simulink model "UserVehicle_RTW"  (Simulink 10.3)
settings: Solver=ode1  StartTime=0.0  StopTime=inf  FixedStep=0.001  RelTol=1e-3
PreLoadFcn:
  | vehicle = 'Car'; if ~length(which('cmcmd')), cmenv; end
  | UserVehicle_RTW_bus
  | UserVehicle_RTW_params
InitFcn:
  | vehicle = 'Car'; if ~length(which('cmcmd')), cmenv; end
  | UserVehicle_RTW_bus
undefined symbols (not defined in the file or in its folder): Car_Bdy1_mass, Car_Steering_i, Car_WhlBaseF, Car_WhlBaseR
libraries: CarMaker4SL x77
(part 3 of 3)

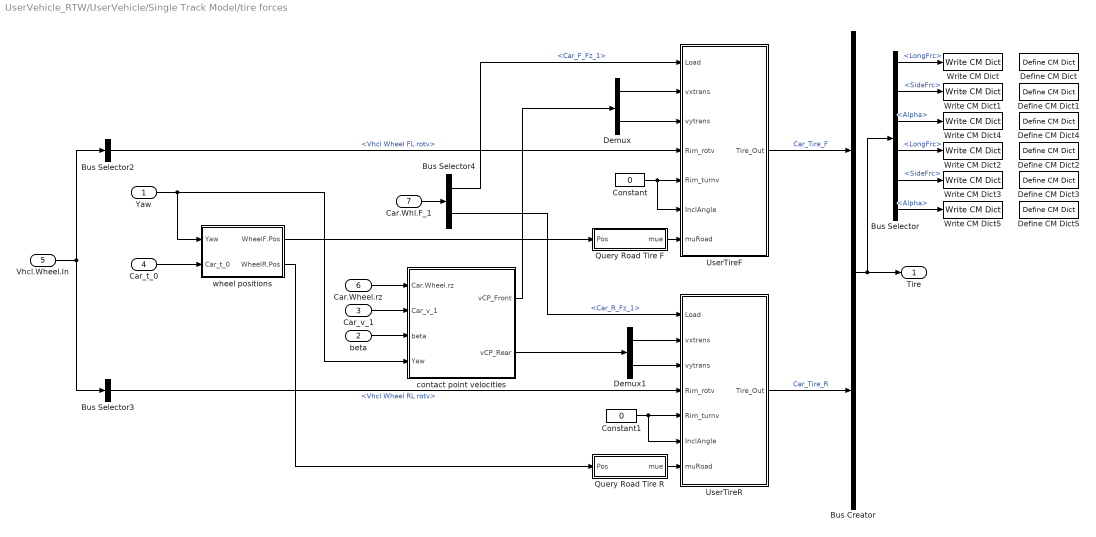
== system UserVehicle_RTW/UserVehicle/Single Track Model/tire forces ==
  Yaw : Inport
  beta : Inport  Port=2
  Car_v_1 : Inport  Port=3
  Car_t_0 : Inport  Port=4
  Vhcl.Wheel.In : Inport  Port=5
  Car.Wheel.rz : Inport  Port=6
  Car.Whl.F_1 : Inport  Port=7
  Bus Creator : BusCreator  Inputs=2
  Bus Selector : BusSelector  OutputSignals=Car_Tire_F.LongFrc,Car_Tire_F.SideFrc,Car_Tire_F.Alpha,Car_Tire_R.LongFrc,Car_Tire_R.SideFrc,Car_Tire_R.Alpha
  Bus Selector2 : BusSelector  OutputSignals=Vhcl Wheel FL rotv
  Bus Selector3 : BusSelector  OutputSignals=Vhcl Wheel RL rotv
  Bus Selector4 : BusSelector  OutputSignals=Car_F_Fz_1,Car_R_Fz_1
  Constant : Constant  Value=0
  Constant1 : Constant  Value=0
  Define CM Dict : CarMaker4SL/Define CM Dict  xname=Tire.F.LongFrc  xunit=N  xmono=off  xtype=Double4  xdvaplace=None  xnstates=0  xfirststate=0  xinitial=0
  Define CM Dict1 : CarMaker4SL/Define CM Dict  xname=Tire.F.SideFrc  xunit=N  xmono=off  xtype=Double4  xdvaplace=None  xnstates=0  xfirststate=0  xinitial=0
  Define CM Dict2 : CarMaker4SL/Define CM Dict  xname=Tire.R.LongFrc  xunit=N  xmono=off  xtype=Double4  xdvaplace=None  xnstates=0  xfirststate=0  xinitial=0
  Define CM Dict3 : CarMaker4SL/Define CM Dict  xname=Tire.R.SideFrc  xunit=N  xmono=off  xtype=Double4  xdvaplace=None  xnstates=0  xfirststate=0  xinitial=0
  Define CM Dict4 : CarMaker4SL/Define CM Dict  xname=Tire.F.Alpha  xunit=rad  xmono=off  xtype=Double4  xdvaplace=None  xnstates=0  xfirststate=0  xinitial=0
  Define CM Dict5 : CarMaker4SL/Define CM Dict  xname=Tire.R.Alpha  xunit=rad  xmono=off  xtype=Double4  xdvaplace=None  xnstates=0  xfirststate=0  xinitial=0
  Demux : Demux  Outputs=2
  Demux1 : Demux  Outputs=2
  Query Road Tire F : Subsystem
  Query Road Tire R : Subsystem
  UserTireF : Subsystem
  UserTireR : Subsystem
  Write CM Dict : CarMaker4SL/Write CM Dict  xname=Tire.F.LongFrc  xsync=off
  Write CM Dict1 : CarMaker4SL/Write CM Dict  xname=Tire.F.SideFrc  xsync=off
  Write CM Dict2 : CarMaker4SL/Write CM Dict  xname=Tire.R.LongFrc  xsync=off
  Write CM Dict3 : CarMaker4SL/Write CM Dict  xname=Tire.R.SideFrc  xsync=off
  Write CM Dict4 : CarMaker4SL/Write CM Dict  xname=Tire.F.Alpha  xsync=off
  Write CM Dict5 : CarMaker4SL/Write CM Dict  xname=Tire.R.Alpha  xsync=off
  contact point velocities : Subsystem
  wheel positions : Subsystem
  Tire : Outport  VectorParamsAs1DForOutWhenUnconnected=off
  wires:
  Bus Selector/6 -> Write CM Dict5/1  "<Alpha>"
  Bus Selector/3 -> Write CM Dict4/1  "<Alpha>"
  Bus Selector/5 -> Write CM Dict3/1  "<SideFrc>"
  Bus Selector/4 -> Write CM Dict2/1  "<LongFrc>"
  Bus Selector/2 -> Write CM Dict1/1  "<SideFrc>"
  Bus Selector/1 -> Write CM Dict/1  "<LongFrc>"
  Demux1/2 -> UserTireR/3(vytrans)
  Demux/2 -> UserTireF/3(vytrans)
  Bus Creator/1 -> Bus Selector/1, Tire/1
  Bus Selector4/1 -> UserTireF/1(Load)  "<Car_F_Fz_1>"
  Car.Whl.F_1/1 -> Bus Selector4/1
  Bus Selector4/2 -> UserTireR/1(Load)  "<Car_R_Fz_1>"
  contact point velocities/2(vCP_Rear) -> Demux1/1
  Demux1/1 -> UserTireR/2(vxtrans)
  Demux/1 -> UserTireF/2(vxtrans)
  contact point velocities/1(vCP_Front) -> Demux/1
  Car.Wheel.rz/1 -> contact point velocities/1(Car.Wheel.rz)
  beta/1 -> contact point velocities/3(beta)
  Car_v_1/1 -> contact point velocities/2(Car_v_1)
  Constant/1 -> UserTireF/5(Rim_turnv), UserTireF/6(InclAngle)
  Bus Selector3/1 -> UserTireR/4(Rim_rotv)  "<Vhcl Wheel RL rotv>"
  wheel positions/2(WheelR.Pos) -> Query Road Tire R/1(Pos)
  wheel positions/1(WheelF.Pos) -> Query Road Tire F/1(Pos)
  Car_t_0/1 -> wheel positions/2(Car_t_0)
  Yaw/1 -> contact point velocities/4(Yaw), wheel positions/1(Yaw)
  Query Road Tire R/1(mue) -> UserTireR/7(muRoad)
  Query Road Tire F/1(mue) -> UserTireF/7(muRoad)
  Bus Selector2/1 -> UserTireF/4(Rim_rotv)  "<Vhcl Wheel FL rotv>"
  Vhcl.Wheel.In/1 -> Bus Selector3/1, Bus Selector2/1
  Constant1/1 -> UserTireR/6(InclAngle), UserTireR/5(Rim_turnv)
  UserTireR/1(Tire_Out) -> Bus Creator/2  "Car_Tire_R"
  UserTireF/1(Tire_Out) -> Bus Creator/1  "Car_Tire_F"

== system UserVehicle_RTW/UserVehicle/Single Track Model/vehicle motion ==
  Car.Whl.F_1 : Inport
  Car.Beta : Inport  Port=2
  Car_Yaw : Inport  Port=3
  global frame : Subsystem
  vehicle frame : Subsystem
  Car.a_1 : Outport  VectorParamsAs1DForOutWhenUnconnected=off
  Car.v_1 : Outport  Port=2  VectorParamsAs1DForOutWhenUnconnected=off
  Car.a_0 : Outport  Port=3  VectorParamsAs1DForOutWhenUnconnected=off
  Car.v_0 : Outport  Port=4  VectorParamsAs1DForOutWhenUnconnected=off
  Car_t_0 : Outport  Port=5  VectorParamsAs1DForOutWhenUnconnected=off
  Car.Dist : Outport  Port=6  VectorParamsAs1DForOutWhenUnconnected=off
  wires:
  global frame/3(Car.t_0) -> Car_t_0/1
  global frame/2(Car_v_0) -> Car.v_0/1
  global frame/1(Car.a_0) -> Car.a_0/1
  Car.Beta/1 -> vehicle frame/2(Car.Beta)
  Car.Whl.F_1/1 -> vehicle frame/1(Car.Whl.F_1)
  vehicle frame/2(Car.v_1) -> global frame/2(Car.v_1), Car.v_1/1
  vehicle frame/1(Car.a_1) -> global frame/1(Car.a_1), Car.a_1/1
  Car_Yaw/1 -> global frame/3(Car.Yaw)
  vehicle frame/3(Car.Dist) -> Car.Dist/1

== system UserVehicle_RTW/UserVehicle/Single Track Model/wheel torques ==
  WheelTrq_1 : Inport
  Add : Sum  Inputs=+-
  Add1 : Sum  Inputs=+-
  Bus Creator : BusCreator  Inputs=2
  Bus Selector1 : BusSelector  OutputSignals=Car_Tire_F.RollResist,Car_Tire_F.LongFrc,Car_Tire_F.rBelt_eff
  Bus Selector2 : BusSelector  OutputSignals=Car_Tire_R.RollResist,Car_Tire_R.LongFrc,Car_Tire_R.rBelt_eff
  Product : Product  RndMeth=Zero
  Product1 : Product  RndMeth=Zero
  Car.Trq2W : Outport  VectorParamsAs1DForOutWhenUnconnected=off
  wires:
  Add1/1 -> Bus Creator/2  "Trq_R"
  Product1/1 -> Add1/2
  Bus Selector2/3 -> Product1/2  "<rBelt_eff>"
  Bus Selector2/2 -> Product1/1  "<LongFrc>"
  Bus Selector2/1 -> Add1/1  "<RollResist>"
  Add/1 -> Bus Creator/1  "Trq_F"
  Product/1 -> Add/2
  Bus Selector1/3 -> Product/2  "<rBelt_eff>"
  Bus Selector1/2 -> Product/1  "<LongFrc>"
  Bus Selector1/1 -> Add/1  "<RollResist>"
  WheelTrq_1/1 -> Bus Selector2/1, Bus Selector1/1
  Bus Creator/1 -> Car.Trq2W/1

== system UserVehicle_RTW/UserVehicle/Single Track Model/yaw ==
  WheelFrc_1 : Inport
  1/ J : Gain  Gain=1/1322.5  SaturateOnIntegerOverflow=on  OutDataTypeStr=Inherit: Same as input  ParamDataTypeStr=Inherit: Same as input
  Bus Creator : BusCreator  Inputs=3
  Bus Selector : BusSelector  OutputSignals=Vhcl Cfg Yaw
  Bus Selector1 : BusSelector  OutputSignals=Car_F_Fy_1,Car_R_Fy_1
  Multiply : Product  Inputs=**  OutDataTypeStr=double
  "S_F * l_F " : Product  InputSameDT=on  SaturateOnIntegerOverflow=on  OutDataTypeStr=Inherit: Same as first input
  "S_R * l_R " : Product  InputSameDT=on  SaturateOnIntegerOverflow=on  OutDataTypeStr=Inherit: Same as first input
  Sum : Sum  Inputs=+-  InputSameDT=on  SaturateOnIntegerOverflow=on  OutDataTypeStr=Inherit: Same as first input
  Vehicle Initial Cfg : CarMaker4SL/Vehicle Initial Cfg
      settings: SourceProductName=CarMaker4SL
  aYaw * dt : Integrator  ExternalReset=level
  l__F : Constant  Value=Car_WhlBaseF
  l__R : Constant  Value=-Car_WhlBaseR
  vYaw * dt : Integrator  ExternalReset=level  InitialConditionSource=external
  Car.Yaw : Outport  VectorParamsAs1DForOutWhenUnconnected=off
  wires:
  Bus Selector1/2 -> "S_R * l_R "/1  "<Car_R_Fy_1>"
  Bus Selector1/1 -> "S_F * l_F "/1  "<Car_F_Fy_1>"
  WheelFrc_1/1 -> Bus Selector1/1
  Bus Creator/1 -> Car.Yaw/1
  "S_R * l_R "/1 -> Sum/2
  l__R/1 -> "S_R * l_R "/2
  "S_F * l_F "/1 -> Sum/1
  l__F/1 -> "S_F * l_F "/2
  Bus Selector/1 -> vYaw * dt/3  "<Vhcl Cfg Yaw>"
  Sum/1 -> 1/ J/1
  1/ J/1 -> Bus Creator/3, aYaw * dt/1  "Yawpp"
  vYaw * dt/1 -> Bus Creator/1  "Yaw"
  Multiply/1 -> Bus Creator/2, vYaw * dt/1  "Yawp"
  [TRStart] -> aYaw * dt/2, vYaw * dt/2
  aYaw * dt/1 -> Multiply/2
  [TRSim] -> Multiply/1
  Vehicle Initial Cfg/1 -> Bus Selector/1

== system UserVehicle_RTW/UserVehicle/CreateBus Vhcl.Fr1/Tr2Fr0/Subsystem_00 ==
  sincos : Inport
  Bus Selector : BusSelector  OutputSignals=cry,crz
  Product : Product  RndMeth=Zero
  Tr2Fr1_00 : Outport  VectorParamsAs1DForOutWhenUnconnected=off
  wires:
  Bus Selector/2 -> Product/2  "<crz>"
  Bus Selector/1 -> Product/1  "<cry>"
  Product/1 -> Tr2Fr1_00/1
  sincos/1 -> Bus Selector/1

== system UserVehicle_RTW/UserVehicle/CreateBus Vhcl.Fr1/Tr2Fr0/Subsystem_01 ==
  sincos : Inport
  Add : Sum  Inputs=+-
  Bus Selector : BusSelector  OutputSignals=srx,sry,crz,crx,srz
  Product : Product  Inputs=3  RndMeth=Zero
  Product1 : Product  RndMeth=Zero
  Tr2Fr1_01 : Outport  VectorParamsAs1DForOutWhenUnconnected=off
  wires:
  Bus Selector/5 -> Product1/2  "<srz>"
  Bus Selector/4 -> Product1/1  "<crx>"
  Bus Selector/3 -> Product/3  "<crz>"
  Bus Selector/2 -> Product/2  "<sry>"
  Bus Selector/1 -> Product/1  "<srx>"
  Add/1 -> Tr2Fr1_01/1
  Product1/1 -> Add/2
  Product/1 -> Add/1
  sincos/1 -> Bus Selector/1

== system UserVehicle_RTW/UserVehicle/CreateBus Vhcl.Fr1/Tr2Fr0/Subsystem_02 ==
  sincos : Inport
  Add : Sum
  Bus Selector : BusSelector  OutputSignals=crx,sry,crz,srx,srz
  Product : Product  Inputs=3  RndMeth=Zero
  Product1 : Product  RndMeth=Zero
  Tr2Fr1_02 : Outport  VectorParamsAs1DForOutWhenUnconnected=off
  wires:
  Bus Selector/4 -> Product1/1  "<srx>"
  Bus Selector/5 -> Product1/2  "<srz>"
  Bus Selector/3 -> Product/3  "<crz>"
  Bus Selector/2 -> Product/2  "<sry>"
  Bus Selector/1 -> Product/1  "<crx>"
  sincos/1 -> Bus Selector/1
  Product/1 -> Add/1
  Product1/1 -> Add/2
  Add/1 -> Tr2Fr1_02/1

== system UserVehicle_RTW/UserVehicle/CreateBus Vhcl.Fr1/Tr2Fr0/Subsystem_10 ==
  sincos : Inport
  Bus Selector : BusSelector  OutputSignals=cry,srz
  Product : Product  RndMeth=Zero
  Tr2Fr1_10 : Outport  VectorParamsAs1DForOutWhenUnconnected=off
  wires:
  sincos/1 -> Bus Selector/1
  Product/1 -> Tr2Fr1_10/1
  Bus Selector/1 -> Product/1  "<cry>"
  Bus Selector/2 -> Product/2  "<srz>"

== system UserVehicle_RTW/UserVehicle/CreateBus Vhcl.Fr1/Tr2Fr0/Subsystem_11 ==
  sincos : Inport
  Add : Sum
  Bus Selector : BusSelector  OutputSignals=srx,sry,srz,crx,crz
  Product : Product  Inputs=3  RndMeth=Zero
  Product1 : Product  RndMeth=Zero
  Tr2Fr1_11 : Outport  VectorParamsAs1DForOutWhenUnconnected=off
  wires:
  Bus Selector/4 -> Product1/1  "<crx>"
  Bus Selector/5 -> Product1/2  "<crz>"
  Bus Selector/3 -> Product/3  "<srz>"
  Bus Selector/2 -> Product/2  "<sry>"
  Bus Selector/1 -> Product/1  "<srx>"
  Add/1 -> Tr2Fr1_11/1
  Product1/1 -> Add/2
  Product/1 -> Add/1
  sincos/1 -> Bus Selector/1

== system UserVehicle_RTW/UserVehicle/CreateBus Vhcl.Fr1/Tr2Fr0/Subsystem_12 ==
  sincos : Inport
  Add : Sum  Inputs=+-
  Bus Selector : BusSelector  OutputSignals=crx,sry,srz,srx,crz
  Product : Product  Inputs=3  RndMeth=Zero
  Product1 : Product  RndMeth=Zero
  Tr2Fr1_12 : Outport  VectorParamsAs1DForOutWhenUnconnected=off
  wires:
  Bus Selector/4 -> Product1/1  "<srx>"
  Bus Selector/5 -> Product1/2  "<crz>"
  Bus Selector/3 -> Product/3  "<srz>"
  Bus Selector/2 -> Product/2  "<sry>"
  Bus Selector/1 -> Product/1  "<crx>"
  sincos/1 -> Bus Selector/1
  Product/1 -> Add/1
  Product1/1 -> Add/2
  Add/1 -> Tr2Fr1_12/1

== system UserVehicle_RTW/UserVehicle/CreateBus Vhcl.Fr1/Tr2Fr0/Subsystem_20 ==
  sincos : Inport
  Bus Selector : BusSelector  OutputSignals=sry
  Gain : Gain  Gain=-1
  Tr2Fr1_20 : Outport  VectorParamsAs1DForOutWhenUnconnected=off
  wires:
  Bus Selector/1 -> Gain/1  "<sry>"
  Gain/1 -> Tr2Fr1_20/1
  sincos/1 -> Bus Selector/1

== system UserVehicle_RTW/UserVehicle/CreateBus Vhcl.Fr1/Tr2Fr0/Subsystem_21 ==
  sincos : Inport
  Bus Selector : BusSelector  OutputSignals=srx,cry
  Product : Product  RndMeth=Zero
  Tr2Fr1_21 : Outport  VectorParamsAs1DForOutWhenUnconnected=off
  wires:
  Bus Selector/2 -> Product/2  "<cry>"
  Bus Selector/1 -> Product/1  "<srx>"
  Product/1 -> Tr2Fr1_21/1
  sincos/1 -> Bus Selector/1

== system UserVehicle_RTW/UserVehicle/CreateBus Vhcl.Fr1/Tr2Fr0/Subsystem_22 ==
  sincos : Inport
  Bus Selector : BusSelector  OutputSignals=crx,cry
  Product : Product  RndMeth=Zero
  Tr2Fr1_22 : Outport  VectorParamsAs1DForOutWhenUnconnected=off
  wires:
  Bus Selector/2 -> Product/2  "<cry>"
  Bus Selector/1 -> Product/1  "<crx>"
  sincos/1 -> Bus Selector/1
  Product/1 -> Tr2Fr1_22/1

== system UserVehicle_RTW/UserVehicle/CreateBus Vhcl.Fr1/Tr2Fr0/sincos ==
  Car : Inport
  Bus Creator : BusCreator  Inputs=6
  Bus Selector : BusSelector  OutputSignals=Road_Fr1_rx,Road_Fr1_ry,Car_Yaw.Yaw
  Trigonometric Function : Trigonometry
  Trigonometric Function1 : Trigonometry  Operator=cos
  Trigonometric Function2 : Trigonometry
  Trigonometric Function3 : Trigonometry
  Trigonometric Function4 : Trigonometry  Operator=cos
  Trigonometric Function5 : Trigonometry  Operator=cos
  sincos : Outport  VectorParamsAs1DForOutWhenUnconnected=off
  wires:
  Bus Creator/1 -> sincos/1
  Trigonometric Function/1 -> Bus Creator/1  "srx"
  Trigonometric Function3/1 -> Bus Creator/2  "sry"
  Trigonometric Function2/1 -> Bus Creator/3  "srz"
  Trigonometric Function1/1 -> Bus Creator/4  "crx"
  Trigonometric Function4/1 -> Bus Creator/5  "cry"
  Trigonometric Function5/1 -> Bus Creator/6  "crz"
  Car/1 -> Bus Selector/1
  Bus Selector/3 -> Trigonometric Function5/1, Trigonometric Function2/1  "<Yaw>"
  Bus Selector/2 -> Trigonometric Function4/1, Trigonometric Function3/1  "<Road_Fr1_ry>"
  Bus Selector/1 -> Trigonometric Function1/1, Trigonometric Function/1  "<Road_Fr1_rx>"

== system UserVehicle_RTW/UserVehicle/Single Track Model/Tire2Wheel/Fr12Fr0_2D ==
  rz : Inport
  x_1 : Inport  Port=2
  y_1 : Inport  Port=3
  Add : Sum  Inputs=+-
  Add1 : Sum
  Demux : Demux  Outputs=2
  Demux1 : Demux  Outputs=2
  Mux : Mux  Inputs=2
  Product : Product  RndMeth=Zero
  Product1 : Product  RndMeth=Zero
  Trigonometric Function : Trigonometry  Operator=cos
  Trigonometric Function1 : Trigonometry
  x_0 : Outport  VectorParamsAs1DForOutWhenUnconnected=off
  y_0 : Outport  Port=2  VectorParamsAs1DForOutWhenUnconnected=off
  wires:
  Trigonometric Function/1 -> Product/1
  Trigonometric Function1/1 -> Product1/1
  Add/1 -> x_0/1
  Add1/1 -> y_0/1
  rz/1 -> Trigonometric Function1/1, Trigonometric Function/1
  x_1/1 -> Mux/1
  y_1/1 -> Mux/2
  Mux/1 -> Product1/2, Product/2
  Product/1 -> Demux/1
  Demux/1 -> Add/1  "x*cos(rz)"
  Product1/1 -> Demux1/1
  Demux1/2 -> Add/2  "y*sin(rz)"
  Demux/2 -> Add1/1  "y*cos(rz)"
  Demux1/1 -> Add1/2  "x*sin(rz)"

== system UserVehicle_RTW/UserVehicle/Single Track Model/sideslip angle/Subsystem ==
  vYaw : Inport
  v : Inport  Port=2
  In3 : Inport  Port=3
  If : If  IfExpression=u1 ~= 0
  If Action Subsystem : Subsystem  TreatAsAtomicUnit=on
  If Action Subsystem1 : Subsystem  TreatAsAtomicUnit=on
  Merge : Merge
  Sum1 : Sum  Inputs=-+  InputSameDT=on  SaturateOnIntegerOverflow=on  OutDataTypeStr=Inherit: Same as first input
  Out1 : Outport  VectorParamsAs1DForOutWhenUnconnected=off
  wires:
  vYaw/1 -> Sum1/1
  v/1 -> If Action Subsystem/1(v), If/1
  Sum1/1 -> Out1/1
  If Action Subsystem/1(Out1) -> Merge/1
  If Action Subsystem1/1(Out1) -> Merge/2
  Merge/1 -> Sum1/2
  If/2 -> If Action Subsystem1/Action
  In3/1 -> If Action Subsystem/2(In3)
  If/1 -> If Action Subsystem/Action

== system UserVehicle_RTW/UserVehicle/Single Track Model/tire forces/Query Road Tire F ==
  Pos : Inport
  Constant1 : Constant  Value=0
  Constant2 : Constant  Value=0
  Define CM Dict1 : CarMaker4SL/Define CM Dict  xname=Tire.F.mue  xmono=off  xtype=Double4  xdvaplace=None  xnstates=0  xfirststate=0  xinitial=0
  Demux : Demux  Outputs=2
  Memory : Memory
  Mux : Mux  Inputs=3
  Subsystem : Subsystem
  Write CM Dict1 : CarMaker4SL/Write CM Dict  xname=Tire.F.mue  xsync=off
  mue : Outport  VectorParamsAs1DForOutWhenUnconnected=off
  wires:
  Constant1/1 -> Subsystem/3(Side)
  [TRSim] -> Subsystem/Enable
  Pos/1 -> Demux/1
  Memory/1 -> Subsystem/2(Dist)
  Demux/1 -> Mux/1
  Demux/2 -> Mux/2
  Mux/1 -> Subsystem/1(xyz)
  Subsystem/2(Dist Out) -> Memory/1
  Subsystem/1(Fric) -> Write CM Dict1/1, mue/1
  Constant2/1 -> Mux/3

== system UserVehicle_RTW/UserVehicle/Single Track Model/tire forces/Query Road Tire R ==
  Pos : Inport
  Constant1 : Constant  Value=0
  Constant2 : Constant  Value=0
  Define CM Dict1 : CarMaker4SL/Define CM Dict  xname=Tire.R.mue  xmono=off  xtype=Double4  xdvaplace=None  xnstates=0  xfirststate=0  xinitial=0
  Demux : Demux  Outputs=2
  Memory : Memory
  Mux : Mux  Inputs=3
  Subsystem : Subsystem
  Write CM Dict1 : CarMaker4SL/Write CM Dict  xname=Tire.R.mue  xsync=off
  mue : Outport  VectorParamsAs1DForOutWhenUnconnected=off
  wires:
  [TRSim] -> Subsystem/Enable
  Constant2/1 -> Mux/3
  Subsystem/1(Fric) -> Write CM Dict1/1, mue/1
  Subsystem/2(Dist Out) -> Memory/1
  Mux/1 -> Subsystem/1(xyz)
  Demux/2 -> Mux/2
  Demux/1 -> Mux/1
  Constant1/1 -> Subsystem/3(Side)
  Memory/1 -> Subsystem/2(Dist)
  Pos/1 -> Demux/1

== system UserVehicle_RTW/UserVehicle/Single Track Model/tire forces/UserTireF ==
  Load : Inport
  vxtrans : Inport  Port=2
  vytrans : Inport  Port=3
  Rim_rotv : Inport  Port=4
  Rim_turnv : Inport  Port=5
  InclAngle : Inport  Port=6
  muRoad : Inport  Port=7
  Bus Creator3 : BusCreator  Inputs=11
  UserTire : S-Function  FunctionName=tire_lin  SFunctionDeploymentMode=off  EnableBusSupport=off
  Tire_Out : Outport  VectorParamsAs1DForOutWhenUnconnected=off
  wires:
  UserTire/8 -> Bus Creator3/8  "LoadFrc"
  UserTire/7 -> Bus Creator3/7  "SideFrc"
  UserTire/6 -> Bus Creator3/6  "LongFrc"
  UserTire/5 -> Bus Creator3/5  "vBelt"
  UserTire/4 -> Bus Creator3/4  "rBelt_eff"
  UserTire/3 -> Bus Creator3/3  "TurnSlp"
  UserTire/2 -> Bus Creator3/2  "Alpha"
  UserTire/1 -> Bus Creator3/1  "Slp"
  Bus Creator3/1 -> Tire_Out/1
  Load/1 -> UserTire/1
  vxtrans/1 -> UserTire/2
  vytrans/1 -> UserTire/3
  Rim_rotv/1 -> UserTire/4
  InclAngle/1 -> UserTire/6
  muRoad/1 -> UserTire/7
  Rim_turnv/1 -> UserTire/5
  UserTire/9 -> Bus Creator3/9  "OverturnTrq"
  UserTire/10 -> Bus Creator3/10  "RollResist"
  UserTire/11 -> Bus Creator3/11  "AlignTrq"

== system UserVehicle_RTW/UserVehicle/Single Track Model/tire forces/UserTireR ==
  Load : Inport
  vxtrans : Inport  Port=2
  vytrans : Inport  Port=3
  Rim_rotv : Inport  Port=4
  Rim_turnv : Inport  Port=5
  InclAngle : Inport  Port=6
  muRoad : Inport  Port=7
  Bus Creator3 : BusCreator  Inputs=11
  UserTire : S-Function  FunctionName=tire_lin  SFunctionDeploymentMode=off  EnableBusSupport=off
  Tire_Out : Outport  VectorParamsAs1DForOutWhenUnconnected=off
  wires:
  UserTire/11 -> Bus Creator3/11  "AlignTrq"
  UserTire/10 -> Bus Creator3/10  "RollResist"
  UserTire/9 -> Bus Creator3/9  "OverturnTrq"
  Rim_turnv/1 -> UserTire/5
  muRoad/1 -> UserTire/7
  InclAngle/1 -> UserTire/6
  Rim_rotv/1 -> UserTire/4
  vytrans/1 -> UserTire/3
  vxtrans/1 -> UserTire/2
  Load/1 -> UserTire/1
  Bus Creator3/1 -> Tire_Out/1
  UserTire/1 -> Bus Creator3/1  "Slp"
  UserTire/2 -> Bus Creator3/2  "Alpha"
  UserTire/3 -> Bus Creator3/3  "TurnSlp"
  UserTire/4 -> Bus Creator3/4  "rBelt_eff"
  UserTire/5 -> Bus Creator3/5  "vBelt"
  UserTire/6 -> Bus Creator3/6  "LongFrc"
  UserTire/7 -> Bus Creator3/7  "SideFrc"
  UserTire/8 -> Bus Creator3/8  "LoadFrc"

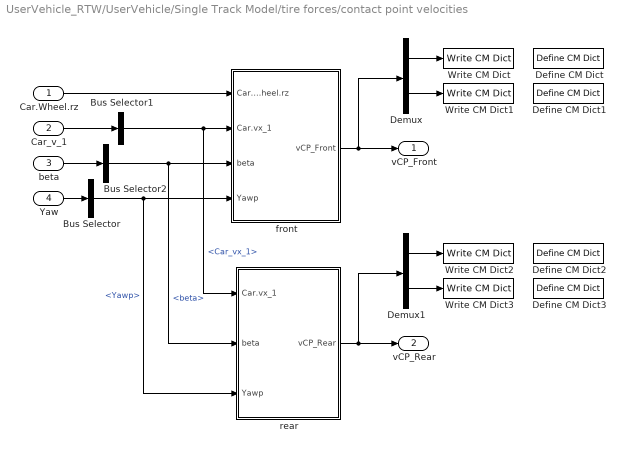
== system UserVehicle_RTW/UserVehicle/Single Track Model/tire forces/contact point velocities ==
  Car.Wheel.rz : Inport
  Car_v_1 : Inport  Port=2
  beta : Inport  Port=3
  Yaw : Inport  Port=4
  Bus Selector : BusSelector  OutputSignals=Yawp
  Bus Selector1 : BusSelector  OutputSignals=Car_vx_1
  Bus Selector2 : BusSelector  OutputSignals=beta
  Define CM Dict : CarMaker4SL/Define CM Dict  xname=Tire.F.vx  xunit=m/s  xmono=off  xtype=Double4  xdvaplace=None  xnstates=0  xfirststate=0  xinitial=0
  Define CM Dict1 : CarMaker4SL/Define CM Dict  xname=Tire.F.vy  xunit=m/s  xmono=off  xtype=Double4  xdvaplace=None  xnstates=0  xfirststate=0  xinitial=0
  Define CM Dict2 : CarMaker4SL/Define CM Dict  xname=Tire.R.vx  xunit=m/s  xmono=off  xtype=Double4  xdvaplace=None  xnstates=0  xfirststate=0  xinitial=0
  Define CM Dict3 : CarMaker4SL/Define CM Dict  xname=Tire.R.vy  xunit=m/s  xmono=off  xtype=Double4  xdvaplace=None  xnstates=0  xfirststate=0  xinitial=0
  Demux : Demux  Outputs=2
  Demux1 : Demux  Outputs=2
  Write CM Dict : CarMaker4SL/Write CM Dict  xname=Tire.F.vx  xsync=off
  Write CM Dict1 : CarMaker4SL/Write CM Dict  xname=Tire.F.vy  xsync=off
  Write CM Dict2 : CarMaker4SL/Write CM Dict  xname=Tire.R.vx  xsync=off
  Write CM Dict3 : CarMaker4SL/Write CM Dict  xname=Tire.R.vy  xsync=off
  front : Subsystem
  rear : Subsystem
  vCP_Front : Outport  VectorParamsAs1DForOutWhenUnconnected=off
  vCP_Rear : Outport  Port=2  VectorParamsAs1DForOutWhenUnconnected=off
  wires:
  Car_v_1/1 -> Bus Selector1/1
  Bus Selector1/1 -> rear/1(Car.vx_1), front/2(Car.vx_1)  "<Car_vx_1>"
  Demux/2 -> Write CM Dict1/1
  Demux/1 -> Write CM Dict/1
  Demux1/2 -> Write CM Dict3/1
  Demux1/1 -> Write CM Dict2/1
  Bus Selector2/1 -> front/3(beta), rear/2(beta)  "<beta>"
  Bus Selector/1 -> rear/3(Yawp), front/4(Yawp)  "<Yawp>"
  Yaw/1 -> Bus Selector/1
  front/1(vCP_Front) -> Demux/1, vCP_Front/1
  Car.Wheel.rz/1 -> front/1(Car.Wheel.rz)
  beta/1 -> Bus Selector2/1
  rear/1(vCP_Rear) -> vCP_Rear/1, Demux1/1

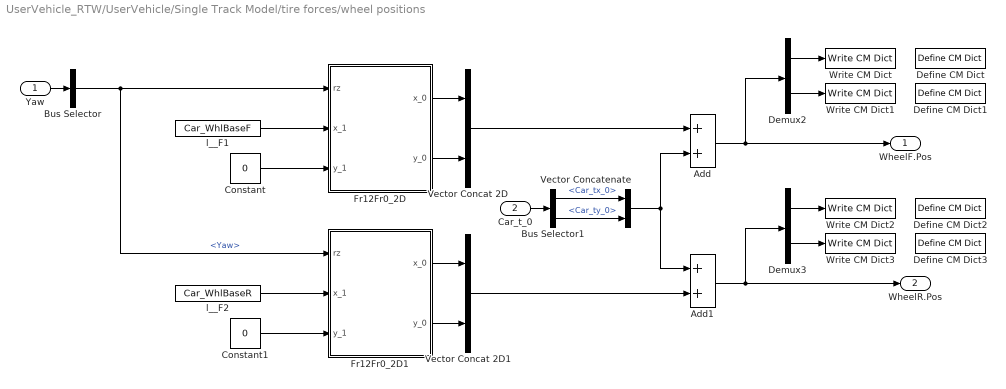
== system UserVehicle_RTW/UserVehicle/Single Track Model/tire forces/wheel positions ==
  Yaw : Inport
  Car_t_0 : Inport  Port=2
  Add : Sum
  Add1 : Sum
  Bus Selector : BusSelector  OutputSignals=Yaw
  Bus Selector1 : BusSelector  OutputSignals=Car_tx_0,Car_ty_0
  Constant : Constant  Value=0
  Constant1 : Constant  Value=0
  Define CM Dict : CarMaker4SL/Define CM Dict  xname=Car.CF.x_0  xunit=m  xmono=off  xtype=Double4  xdvaplace=None  xnstates=0  xfirststate=0  xinitial=0
  Define CM Dict1 : CarMaker4SL/Define CM Dict  xname=Car.CF.y_0  xunit=m  xmono=off  xtype=Double4  xdvaplace=None  xnstates=0  xfirststate=0  xinitial=0
  Define CM Dict2 : CarMaker4SL/Define CM Dict  xname=Car.CR.x_0  xunit=m  xmono=off  xtype=Double4  xdvaplace=None  xnstates=0  xfirststate=0  xinitial=0
  Define CM Dict3 : CarMaker4SL/Define CM Dict  xname=Car.CR.y_0  xunit=m  xmono=off  xtype=Double4  xdvaplace=None  xnstates=0  xfirststate=0  xinitial=0
  Demux2 : Demux  Outputs=2
  Demux3 : Demux  Outputs=2
  Fr12Fr0_2D : Subsystem
  Fr12Fr0_2D1 : Subsystem
  Vector Concat 2D : Concatenate
  Vector Concat 2D1 : Concatenate
  Vector Concatenate : Concatenate
  Write CM Dict : CarMaker4SL/Write CM Dict  xname=Car.CF.x_0  xsync=off
  Write CM Dict1 : CarMaker4SL/Write CM Dict  xname=Car.CF.y_0  xsync=off
  Write CM Dict2 : CarMaker4SL/Write CM Dict  xname=Car.CR.x_0  xsync=off
  Write CM Dict3 : CarMaker4SL/Write CM Dict  xname=Car.CR.y_0  xsync=off
  l__F1 : Constant  Value=Car_WhlBaseF
  l__F2 : Constant  Value=Car_WhlBaseR
  WheelF.Pos : Outport  VectorParamsAs1DForOutWhenUnconnected=off
  WheelR.Pos : Outport  Port=2  VectorParamsAs1DForOutWhenUnconnected=off
  wires:
  Bus Selector1/2 -> Vector Concatenate/2  "<Car_ty_0>"
  Bus Selector1/1 -> Vector Concatenate/1  "<Car_tx_0>"
  Vector Concatenate/1 -> Add1/1, Add/2
  Car_t_0/1 -> Bus Selector1/1
  Add1/1 -> Demux3/1, WheelR.Pos/1
  Vector Concat 2D1/1 -> Add1/2
  Add/1 -> Demux2/1, WheelF.Pos/1
  Vector Concat 2D/1 -> Add/1
  Constant1/1 -> Fr12Fr0_2D1/3(y_1)
  Constant/1 -> Fr12Fr0_2D/3(y_1)
  Demux3/2 -> Write CM Dict3/1
  Demux3/1 -> Write CM Dict2/1
  Demux2/2 -> Write CM Dict1/1
  Demux2/1 -> Write CM Dict/1
  Bus Selector/1 -> Fr12Fr0_2D1/1(rz), Fr12Fr0_2D/1(rz)  "<Yaw>"
  Yaw/1 -> Bus Selector/1
  Fr12Fr0_2D1/2(y_0) -> Vector Concat 2D1/2
  Fr12Fr0_2D1/1(x_0) -> Vector Concat 2D1/1
  Fr12Fr0_2D/2(y_0) -> Vector Concat 2D/2
  Fr12Fr0_2D/1(x_0) -> Vector Concat 2D/1
  l__F2/1 -> Fr12Fr0_2D1/2(x_1)
  l__F1/1 -> Fr12Fr0_2D/2(x_1)

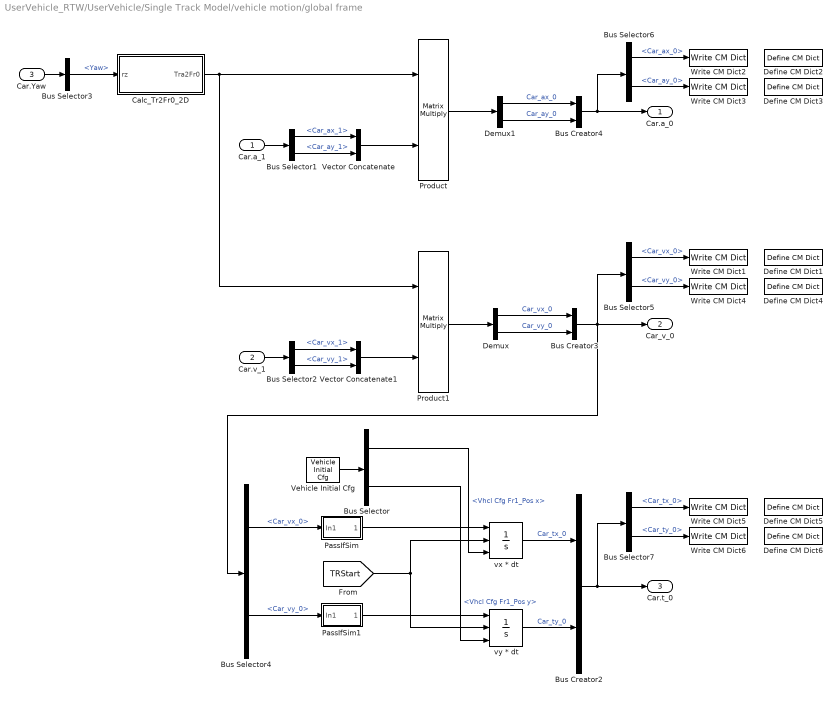
== system UserVehicle_RTW/UserVehicle/Single Track Model/vehicle motion/global frame ==
  Car.a_1 : Inport
  Car.v_1 : Inport  Port=2
  Car.Yaw : Inport  Port=3
  Bus Creator2 : BusCreator  Inputs=2
  Bus Creator3 : BusCreator  Inputs=2
  Bus Creator4 : BusCreator  Inputs=2
  Bus Selector : BusSelector  OutputSignals=Vhcl Cfg Fr1_Pos x,Vhcl Cfg Fr1_Pos y
  Bus Selector1 : BusSelector  OutputSignals=Car_ax_1,Car_ay_1
  Bus Selector2 : BusSelector  OutputSignals=Car_vx_1,Car_vy_1
  Bus Selector3 : BusSelector  OutputSignals=Yaw
  Bus Selector4 : BusSelector  OutputSignals=Car_vx_0,Car_vy_0
  Bus Selector5 : BusSelector  OutputSignals=Car_vx_0,Car_vy_0
  Bus Selector6 : BusSelector  OutputSignals=Car_ax_0,Car_ay_0
  Bus Selector7 : BusSelector  OutputSignals=Car_tx_0,Car_ty_0
  Calc_Tr2Fr0_2D : Subsystem
  Define CM Dict1 : CarMaker4SL/Define CM Dict  xname=Car.vx_0  xunit=m/s  xmono=off  xtype=Double4  xdvaplace=None  xnstates=0  xfirststate=0  xinitial=0
  Define CM Dict2 : CarMaker4SL/Define CM Dict  xname=Car.ax_0  xunit=m/s^2  xmono=off  xtype=Double4  xdvaplace=None  xnstates=0  xfirststate=0  xinitial=0
  Define CM Dict3 : CarMaker4SL/Define CM Dict  xname=Car.ay_0  xunit=m/s^2  xmono=off  xtype=Double4  xdvaplace=None  xnstates=0  xfirststate=0  xinitial=0
  Define CM Dict4 : CarMaker4SL/Define CM Dict  xname=Car.vy_0  xunit=m/s  xmono=off  xtype=Double4  xdvaplace=None  xnstates=0  xfirststate=0  xinitial=0
  Define CM Dict5 : CarMaker4SL/Define CM Dict  xname=Car.tx_0  xunit=m  xmono=off  xtype=Double4  xdvaplace=None  xnstates=0  xfirststate=0  xinitial=0
  Define CM Dict6 : CarMaker4SL/Define CM Dict  xname=Car.ty_0  xunit=m  xmono=off  xtype=Double4  xdvaplace=None  xnstates=0  xfirststate=0  xinitial=0
  Demux : Demux  Outputs=2
  Demux1 : Demux  Outputs=2
  PassIfSim : Subsystem
  PassIfSim1 : Subsystem
  Product : Product  Multiplication=Matrix(*)  RndMeth=Zero
  Product1 : Product  Multiplication=Matrix(*)  RndMeth=Zero
  Vector Concatenate : Concatenate
  Vector Concatenate1 : Concatenate
  Vehicle Initial Cfg : CarMaker4SL/Vehicle Initial Cfg
      settings: SourceProductName=CarMaker4SL
  Write CM Dict1 : CarMaker4SL/Write CM Dict  xname=Car.vx_0  xsync=off
  Write CM Dict2 : CarMaker4SL/Write CM Dict  xname=Car.ax_0  xsync=off
  Write CM Dict3 : CarMaker4SL/Write CM Dict  xname=Car.ay_0  xsync=off
  Write CM Dict4 : CarMaker4SL/Write CM Dict  xname=Car.vy_0  xsync=off
  Write CM Dict5 : CarMaker4SL/Write CM Dict  xname=Car.tx_0  xsync=off
  Write CM Dict6 : CarMaker4SL/Write CM Dict  xname=Car.ty_0  xsync=off
  vx * dt : Integrator  ExternalReset=level  InitialConditionSource=external  InitialCondition=[0,0]
  vy * dt : Integrator  ExternalReset=level  InitialConditionSource=external  InitialCondition=[0,0]
  Car.a_0 : Outport  VectorParamsAs1DForOutWhenUnconnected=off
  Car_v_0 : Outport  Port=2  VectorParamsAs1DForOutWhenUnconnected=off
  Car.t_0 : Outport  Port=3  VectorParamsAs1DForOutWhenUnconnected=off
  wires:
  Bus Selector3/1 -> Calc_Tr2Fr0_2D/1(rz)  "<Yaw>"
  Bus Selector7/2 -> Write CM Dict6/1  "<Car_ty_0>"
  Bus Selector7/1 -> Write CM Dict5/1  "<Car_tx_0>"
  Bus Selector6/2 -> Write CM Dict3/1  "<Car_ay_0>"
  Bus Selector6/1 -> Write CM Dict2/1  "<Car_ax_0>"
  Bus Selector5/2 -> Write CM Dict4/1  "<Car_vy_0>"
  Bus Selector5/1 -> Write CM Dict1/1  "<Car_vx_0>"
  Vector Concatenate1/1 -> Product1/2
  Bus Selector2/2 -> Vector Concatenate1/2  "<Car_vy_1>"
  Bus Selector2/1 -> Vector Concatenate1/1  "<Car_vx_1>"
  Vector Concatenate/1 -> Product/2
  Bus Selector1/2 -> Vector Concatenate/2  "<Car_ay_1>"
  Bus Selector1/1 -> Vector Concatenate/1  "<Car_ax_1>"
  Car.v_1/1 -> Bus Selector2/1
  Car.a_1/1 -> Bus Selector1/1
  Bus Creator4/1 -> Bus Selector6/1, Car.a_0/1
  Car.Yaw/1 -> Bus Selector3/1
  Bus Creator2/1 -> Bus Selector7/1, Car.t_0/1
  Product/1 -> Demux1/1
  Demux1/2 -> Bus Creator4/2  "Car_ay_0"
  Demux1/1 -> Bus Creator4/1  "Car_ax_0"
  Bus Creator3/1 -> Bus Selector5/1, Bus Selector4/1, Car_v_0/1
  Demux/2 -> Bus Creator3/2  "Car_vy_0"
  Demux/1 -> Bus Creator3/1  "Car_vx_0"
  Product1/1 -> Demux/1
  Calc_Tr2Fr0_2D/1(Tra2Fr0) -> Product/1, Product1/1
  PassIfSim1/1(Out1) -> vy * dt/1
  Bus Selector4/2 -> PassIfSim1/1(In1)  "<Car_vy_0>"
  PassIfSim/1(Out1) -> vx * dt/1
  Bus Selector4/1 -> PassIfSim/1(In1)  "<Car_vx_0>"
  [TRStart] -> vx * dt/2, vy * dt/2
  vy * dt/1 -> Bus Creator2/2  "Car_ty_0"
  vx * dt/1 -> Bus Creator2/1  "Car_tx_0"
  Vehicle Initial Cfg/1 -> Bus Selector/1
  Bus Selector/2 -> vy * dt/3  "<Vhcl Cfg Fr1_Pos y>"
  Bus Selector/1 -> vx * dt/3  "<Vhcl Cfg Fr1_Pos x>"

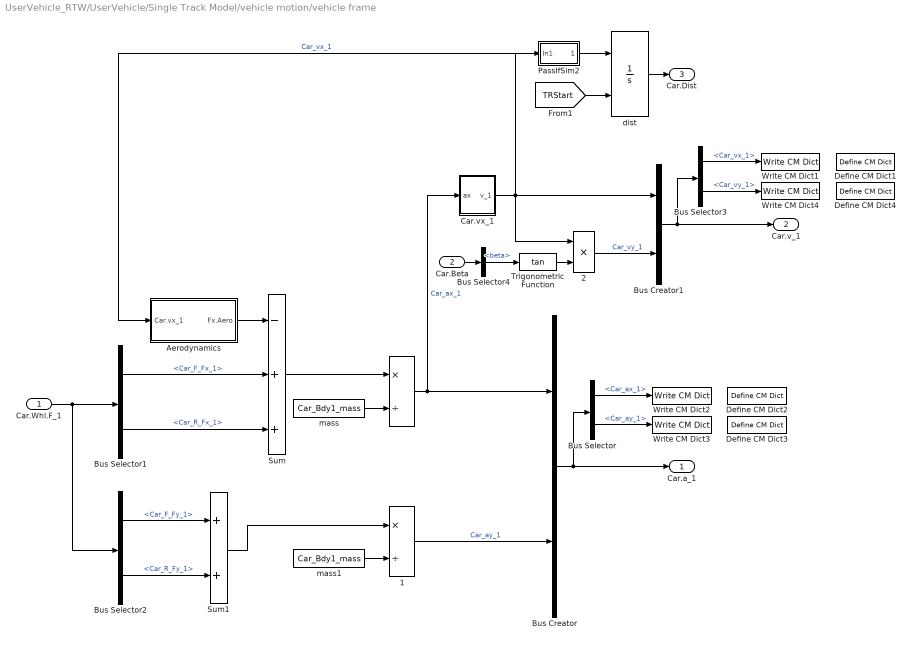
== system UserVehicle_RTW/UserVehicle/Single Track Model/vehicle motion/vehicle frame ==
  Car.Whl.F_1 : Inport
  Car.Beta : Inport  Port=2
  "      " : Product  Inputs=*/  InputSameDT=on  SaturateOnIntegerOverflow=on  OutDataTypeStr=Inherit: Same as first input
  "      1" : Product  Inputs=*/  InputSameDT=on  SaturateOnIntegerOverflow=on  OutDataTypeStr=Inherit: Same as first input
  "      2" : Product  Inputs=**  InputSameDT=on  SaturateOnIntegerOverflow=on  OutDataTypeStr=Inherit: Same as first input
  Aerodynamics : Subsystem
  Bus Creator : BusCreator  Inputs=2
  Bus Creator1 : BusCreator  Inputs=2
  Bus Selector : BusSelector  OutputSignals=Car_ax_1,Car_ay_1
  Bus Selector1 : BusSelector  OutputSignals=Car_F_Fx_1,Car_R_Fx_1
  Bus Selector2 : BusSelector  OutputSignals=Car_F_Fy_1,Car_R_Fy_1
  Bus Selector3 : BusSelector  OutputSignals=Car_vx_1,Car_vy_1
  Bus Selector4 : BusSelector  OutputSignals=beta
  Car.vx_1 : Subsystem
  Define CM Dict1 : CarMaker4SL/Define CM Dict  xname=Car.vx_1  xunit=m/s  xmono=off  xtype=Double4  xdvaplace=None  xnstates=0  xfirststate=0  xinitial=0
  Define CM Dict2 : CarMaker4SL/Define CM Dict  xname=Car.ax_1  xunit=m/s^2  xmono=off  xtype=Double4  xdvaplace=None  xnstates=0  xfirststate=0  xinitial=0
  Define CM Dict3 : CarMaker4SL/Define CM Dict  xname=Car.ay_1  xunit=m/s^2  xmono=off  xtype=Double4  xdvaplace=None  xnstates=0  xfirststate=0  xinitial=0
  Define CM Dict4 : CarMaker4SL/Define CM Dict  xname=Car.vy_1  xunit=m/s  xmono=off  xtype=Double4  xdvaplace=None  xnstates=0  xfirststate=0  xinitial=0
  PassIfSim2 : Subsystem
  Sum : Sum  Inputs=-++  InputSameDT=on  SaturateOnIntegerOverflow=on  OutDataTypeStr=Inherit: Same as first input
  Sum1 : Sum  InputSameDT=on  SaturateOnIntegerOverflow=on  OutDataTypeStr=Inherit: Same as first input
  Trigonometric Function : Trigonometry  Operator=tan
  Write CM Dict1 : CarMaker4SL/Write CM Dict  xname=Car.vx_1  xsync=off
  Write CM Dict2 : CarMaker4SL/Write CM Dict  xname=Car.ax_1  xsync=off
  Write CM Dict3 : CarMaker4SL/Write CM Dict  xname=Car.ay_1  xsync=off
  Write CM Dict4 : CarMaker4SL/Write CM Dict  xname=Car.vy_1  xsync=off
  dist : Integrator  ExternalReset=level
  mass : Constant  Value=Car_Bdy1_mass
  mass1 : Constant  Value=Car_Bdy1_mass
  Car.a_1 : Outport  VectorParamsAs1DForOutWhenUnconnected=off
  Car.v_1 : Outport  Port=2  VectorParamsAs1DForOutWhenUnconnected=off
  Car.Dist : Outport  Port=3  VectorParamsAs1DForOutWhenUnconnected=off
  wires:
  Bus Selector4/1 -> Trigonometric Function/1  "<beta>"
  Car.Beta/1 -> Bus Selector4/1
  Trigonometric Function/1 -> "      2"/2
  "      2"/1 -> Bus Creator1/2  "Car_vy_1"
  Bus Selector2/2 -> Sum1/2  "<Car_R_Fy_1>"
  Bus Selector2/1 -> Sum1/1  "<Car_F_Fy_1>"
  mass1/1 -> "      1"/2
  Sum1/1 -> "      1"/1
  Bus Selector3/2 -> Write CM Dict4/1  "<Car_vy_1>"
  Bus Selector3/1 -> Write CM Dict1/1  "<Car_vx_1>"
  Bus Selector/2 -> Write CM Dict3/1  "<Car_ay_1>"
  Bus Selector/1 -> Write CM Dict2/1  "<Car_ax_1>"
  dist/1 -> Car.Dist/1
  Bus Creator1/1 -> Bus Selector3/1, Car.v_1/1
  Aerodynamics/1(Fx.Aero) -> Sum/1
  Bus Creator/1 -> Bus Selector/1, Car.a_1/1
  "      1"/1 -> Bus Creator/2  "Car_ay_1"
  Bus Selector1/2 -> Sum/3  "<Car_R_Fx_1>"
  [TRStart] -> dist/2
  PassIfSim2/1(Out1) -> dist/1
  Bus Selector1/1 -> Sum/2  "<Car_F_Fx_1>"
  Car.Whl.F_1/1 -> Bus Selector2/1, Bus Selector1/1
  Car.vx_1/1(v_1) -> "      2"/1, Bus Creator1/1, PassIfSim2/1(In1), Aerodynamics/1(Car.vx_1)  "Car_vx_1"
  mass/1 -> "      "/2
  "      "/1 -> Bus Creator/1, Car.vx_1/1(ax)  "Car_ax_1"
  Sum/1 -> "      "/1

== system UserVehicle_RTW/UserVehicle/Single Track Model/sideslip angle/Subsystem/If Action Subsystem ==
  v : Inport
  In3 : Inport  Port=2
  Action Port : ActionPort  ActionPortLabel=if { }
  "    " : Product  Inputs=/*  InputSameDT=on  SaturateOnIntegerOverflow=on  OutDataTypeStr=Inherit: Same as first input
  Out1 : Outport  InitialOutput=0  VectorParamsAs1DForOutWhenUnconnected=off
  wires:
  v/1 -> "    "/1
  In3/1 -> "    "/2
  "    "/1 -> Out1/1

== system UserVehicle_RTW/UserVehicle/Single Track Model/sideslip angle/Subsystem/If Action Subsystem1 ==
  Action Port : ActionPort  ActionPortLabel=else { }
  Constant : Constant  Value=0
  Out1 : Outport  InitialOutput=0  VectorParamsAs1DForOutWhenUnconnected=off
  wires:
  Constant/1 -> Out1/1

== system UserVehicle_RTW/UserVehicle/Single Track Model/tire forces/Query Road Tire F/Subsystem ==
  xyz : Inport
  Dist : Inport  Port=2
  Side : Inport  Port=3
  Enable : EnablePort
  Bus Selector2 : BusSelector  OutputSignals=fric,s
  IPGRoad5 : CarMaker4SL/IPGRoad5  xname=IPGRoad  xevalmode=RouteEval XY_S  xconsiderbumps=off  xusepath=off  xwithcurve=off  xabort=on
      settings: SourceProductName=CarMaker4SL
  Mux : Mux  Inputs=2
  Terminator : Terminator
  Fric : Outport  VectorParamsAs1DForOutWhenUnconnected=off
  Dist Out : Outport  Port=2  VectorParamsAs1DForOutWhenUnconnected=off
  wires:
  Bus Selector2/1 -> Fric/1  "<fric>"
  Bus Selector2/2 -> Dist Out/1  "<s>"
  Mux/1 -> IPGRoad5/1
  IPGRoad5/1 -> Terminator/1
  Side/1 -> Mux/2
  IPGRoad5/2 -> Bus Selector2/1
  Dist/1 -> Mux/1
  xyz/1 -> IPGRoad5/2

== system UserVehicle_RTW/UserVehicle/Single Track Model/tire forces/Query Road Tire R/Subsystem ==
  xyz : Inport
  Dist : Inport  Port=2
  Side : Inport  Port=3
  Enable : EnablePort
  Bus Selector2 : BusSelector  OutputSignals=fric,s
  IPGRoad5 : CarMaker4SL/IPGRoad5  xname=IPGRoad  xevalmode=RouteEval ST  xconsiderbumps=off  xusepath=off  xwithcurve=off  xabort=on
      settings: SourceProductName=CarMaker4SL
  Mux : Mux  Inputs=2
  Terminator : Terminator
  Fric : Outport  VectorParamsAs1DForOutWhenUnconnected=off
  Dist Out : Outport  Port=2  VectorParamsAs1DForOutWhenUnconnected=off
  wires:
  IPGRoad5/2 -> Bus Selector2/1
  Bus Selector2/1 -> Fric/1  "<fric>"
  Bus Selector2/2 -> Dist Out/1  "<s>"
  IPGRoad5/1 -> Terminator/1
  Mux/1 -> IPGRoad5/1
  Side/1 -> Mux/2
  Dist/1 -> Mux/1
  xyz/1 -> IPGRoad5/2

== system UserVehicle_RTW/UserVehicle/Single Track Model/tire forces/contact point velocities/front ==
  Car.Wheel.rz : Inport
  Car.vx_1 : Inport  Port=2
  beta : Inport  Port=3
  Yawp : Inport  Port=4
  Add : Sum
  Calc_Tr2FrW_2D : Subsystem
  Product : Product  RndMeth=Zero
  Product1 : Product  RndMeth=Zero
  Product2 : Product  RndMeth=Zero
  Product3 : Product  Multiplication=Matrix(*)  RndMeth=Zero
  Vector Concatenate : Concatenate
  cos(beta) : Trigonometry  Operator=cos
  l__F2 : Constant  Value=Car_WhlBaseF
  sin(beta) : Trigonometry
  vCP_Front : Outport  VectorParamsAs1DForOutWhenUnconnected=off
  wires:
  Product3/1 -> vCP_Front/1
  beta/1 -> sin(beta)/1, cos(beta)/1
  Calc_Tr2FrW_2D/1(Tra2FrW) -> Product3/1
  Vector Concatenate/1 -> Product3/2
  Car.Wheel.rz/1 -> Calc_Tr2FrW_2D/1(rz)
  Add/1 -> Vector Concatenate/2  "vy"
  Product/1 -> Vector Concatenate/1  "vx"
  cos(beta)/1 -> Product/2
  Car.vx_1/1 -> Product/1, Product1/1
  sin(beta)/1 -> Product1/2
  Product1/1 -> Add/1
  Product2/1 -> Add/2
  l__F2/1 -> Product2/2
  Yawp/1 -> Product2/1

== system UserVehicle_RTW/UserVehicle/Single Track Model/tire forces/contact point velocities/rear ==
  Car.vx_1 : Inport
  beta : Inport  Port=2
  Yawp : Inport  Port=3
  Add : Sum  Inputs=+-
  Product : Product  RndMeth=Zero
  Product1 : Product  RndMeth=Zero
  Product2 : Product  RndMeth=Zero
  Vector Concatenate : Concatenate
  cos(beta) : Trigonometry  Operator=cos
  l__F2 : Constant  Value=-Car_WhlBaseR
  sin(beta) : Trigonometry
  vCP_Rear : Outport  VectorParamsAs1DForOutWhenUnconnected=off
  wires:
  Yawp/1 -> Product2/1
  Vector Concatenate/1 -> vCP_Rear/1
  l__F2/1 -> Product2/2
  Product2/1 -> Add/2
  Product1/1 -> Add/1
  sin(beta)/1 -> Product1/2
  Car.vx_1/1 -> Product1/1, Product/1
  cos(beta)/1 -> Product/2
  Product/1 -> Vector Concatenate/1  "vx"
  Add/1 -> Vector Concatenate/2  "vy"
  beta/1 -> sin(beta)/1, cos(beta)/1

== system UserVehicle_RTW/UserVehicle/Single Track Model/tire forces/wheel positions/Fr12Fr0_2D ==
  rz : Inport
  x_1 : Inport  Port=2
  y_1 : Inport  Port=3
  Add : Sum  Inputs=+-
  Add1 : Sum
  Demux : Demux  Outputs=2
  Demux1 : Demux  Outputs=2
  Mux : Mux  Inputs=2
  Product : Product  RndMeth=Zero
  Product1 : Product  RndMeth=Zero
  Trigonometric Function : Trigonometry  Operator=cos
  Trigonometric Function1 : Trigonometry
  x_0 : Outport  VectorParamsAs1DForOutWhenUnconnected=off
  y_0 : Outport  Port=2  VectorParamsAs1DForOutWhenUnconnected=off
  wires:
  Trigonometric Function/1 -> Product/1
  Trigonometric Function1/1 -> Product1/1
  Add/1 -> x_0/1
  Add1/1 -> y_0/1
  rz/1 -> Trigonometric Function1/1, Trigonometric Function/1
  x_1/1 -> Mux/1
  y_1/1 -> Mux/2
  Mux/1 -> Product1/2, Product/2
  Product/1 -> Demux/1
  Demux/1 -> Add/1  "x*cos(rz)"
  Product1/1 -> Demux1/1
  Demux1/2 -> Add/2  "y*sin(rz)"
  Demux/2 -> Add1/1  "y*cos(rz)"
  Demux1/1 -> Add1/2  "x*sin(rz)"

== system UserVehicle_RTW/UserVehicle/Single Track Model/tire forces/wheel positions/Fr12Fr0_2D1 ==
  rz : Inport
  x_1 : Inport  Port=2
  y_1 : Inport  Port=3
  Add : Sum  Inputs=+-
  Add1 : Sum
  Demux : Demux  Outputs=2
  Demux1 : Demux  Outputs=2
  Mux : Mux  Inputs=2
  Product : Product  RndMeth=Zero
  Product1 : Product  RndMeth=Zero
  Trigonometric Function : Trigonometry  Operator=cos
  Trigonometric Function1 : Trigonometry
  x_0 : Outport  VectorParamsAs1DForOutWhenUnconnected=off
  y_0 : Outport  Port=2  VectorParamsAs1DForOutWhenUnconnected=off
  wires:
  Trigonometric Function/1 -> Product/1
  Trigonometric Function1/1 -> Product1/1
  Add/1 -> x_0/1
  Add1/1 -> y_0/1
  rz/1 -> Trigonometric Function1/1, Trigonometric Function/1
  x_1/1 -> Mux/1
  y_1/1 -> Mux/2
  Mux/1 -> Product1/2, Product/2
  Product/1 -> Demux/1
  Demux/1 -> Add/1  "x*cos(rz)"
  Product1/1 -> Demux1/1
  Demux1/2 -> Add/2  "y*sin(rz)"
  Demux/2 -> Add1/1  "y*cos(rz)"
  Demux1/1 -> Add1/2  "x*sin(rz)"

== system UserVehicle_RTW/UserVehicle/Single Track Model/vehicle motion/global frame/Calc_Tr2Fr0_2D ==
  rz : Inport
  Create 2x2 Matrix : Subsystem
  Gain : Gain  Gain=-1
  Trigonometric Function : Trigonometry  Operator=cos
  Trigonometric Function1 : Trigonometry
  Tra2Fr0 : Outport  VectorParamsAs1DForOutWhenUnconnected=off
  wires:
  Create 2x2 Matrix/1(A) -> Tra2Fr0/1  "Tra2Fr0"
  rz/1 -> Trigonometric Function/1, Trigonometric Function1/1
  Trigonometric Function/1 -> Create 2x2 Matrix/1(A00), Create 2x2 Matrix/4(A11)
  Trigonometric Function1/1 -> Gain/1, Create 2x2 Matrix/3(A10)
  Gain/1 -> Create 2x2 Matrix/2(A01)

== system UserVehicle_RTW/UserVehicle/Single Track Model/vehicle motion/global frame/PassIfSim ==
  note: Output original value only when simulating,
      | and zero during pre- or postprocessing.
  In1 : Inport
  "   " : Product  InputSameDT=on  SaturateOnIntegerOverflow=on  OutDataTypeStr=Inherit: Same as first input
  Data Type Conversion : DataTypeConversion
  Out1 : Outport  VectorParamsAs1DForOutWhenUnconnected=off
  wires:
  In1/1 -> "   "/1
  Data Type Conversion/1 -> "   "/2
  "   "/1 -> Out1/1
  [TRSim] -> Data Type Conversion/1

== system UserVehicle_RTW/UserVehicle/Single Track Model/vehicle motion/global frame/PassIfSim1 ==
  note: Output original value only when simulating,
      | and zero during pre- or postprocessing.
  In1 : Inport
  "   " : Product  InputSameDT=on  SaturateOnIntegerOverflow=on  OutDataTypeStr=Inherit: Same as first input
  Data Type Conversion : DataTypeConversion
  Out1 : Outport  VectorParamsAs1DForOutWhenUnconnected=off
  wires:
  In1/1 -> "   "/1
  Data Type Conversion/1 -> "   "/2
  "   "/1 -> Out1/1
  [TRSim] -> Data Type Conversion/1

== system UserVehicle_RTW/UserVehicle/Single Track Model/vehicle motion/vehicle frame/Aerodynamics ==
  Car.vx_1 : Inport
  A : Constant  Value=1.7
  Constant6 : Constant  Value=0.5
  Product3 : Product  Inputs=5  InputSameDT=on  SaturateOnIntegerOverflow=on  OutDataTypeStr=Inherit: Same as first input
  Product4 : Product  InputSameDT=on  SaturateOnIntegerOverflow=on  OutDataTypeStr=Inherit: Same as first input
  cW : Constant  Value=0.5
  rho : Constant  Value=1.205
  Fx.Aero : Outport  VectorParamsAs1DForOutWhenUnconnected=off
  wires:
  Product3/1 -> Fx.Aero/1
  Car.vx_1/1 -> Product4/2, Product4/1
  A/1 -> Product3/5
  rho/1 -> Product3/4
  Constant6/1 -> Product3/3
  cW/1 -> Product3/2
  Product4/1 -> Product3/1

== system UserVehicle_RTW/UserVehicle/Single Track Model/vehicle motion/vehicle frame/Car.vx_1 ==
  ax : Inport
  Constant1 : Constant  Value=0.1
  PassIfSim : Subsystem
  Read CM Parameter : CarMaker4SL/Read CM Parameter  xfile=Testrun  xkey=DrivMan.Man.Start.Velocity  xnout=1  xdefaults=0  xmuxed=on
      settings: SourceProductName=CarMaker4SL
  kmh2ms : Gain  Gain=1000/3600  OutDataTypeStr=Inherit: Inherit via back propagation  SaturateOnIntegerOverflow=on  ParamDataTypeStr=Inherit: Same as input
  vMin : MinMax  Function=max  Inputs=2  InputSameDT=on  SaturateOnIntegerOverflow=on
  v_dot * dt : Integrator  ExternalReset=level  InitialConditionSource=external  InitialCondition=22.222
  v_1 : Outport  VectorParamsAs1DForOutWhenUnconnected=off
  wires:
  PassIfSim/1(Out1) -> v_dot * dt/1
  ax/1 -> PassIfSim/1(In1)
  v_dot * dt/1 -> v_1/1
  vMin/1 -> v_dot * dt/3
  [TRStart] -> v_dot * dt/2
  Constant1/1 -> vMin/1
  kmh2ms/1 -> vMin/2
  Read CM Parameter/1 -> kmh2ms/1

== system UserVehicle_RTW/UserVehicle/Single Track Model/vehicle motion/vehicle frame/PassIfSim2 ==
  note: Output original value only when simulating,
      | and zero during pre- or postprocessing.
  In1 : Inport
  "   " : Product  InputSameDT=on  SaturateOnIntegerOverflow=on  OutDataTypeStr=Inherit: Same as first input
  Data Type Conversion : DataTypeConversion
  Out1 : Outport  VectorParamsAs1DForOutWhenUnconnected=off
  wires:
  In1/1 -> "   "/1
  Data Type Conversion/1 -> "   "/2
  "   "/1 -> Out1/1
  [TRSim] -> Data Type Conversion/1

== system UserVehicle_RTW/UserVehicle/Single Track Model/tire forces/contact point velocities/front/Calc_Tr2FrW_2D ==
  rz : Inport
  Create 2x2 Matrix : Subsystem
  Gain : Gain  Gain=-1
  Trigonometric Function : Trigonometry  Operator=cos
  Trigonometric Function1 : Trigonometry
  Tra2FrW : Outport  VectorParamsAs1DForOutWhenUnconnected=off
  wires:
  Gain/1 -> Create 2x2 Matrix/3(A10)
  Create 2x2 Matrix/1(A) -> Tra2FrW/1  "Tra2FrW"
  rz/1 -> Trigonometric Function/1, Trigonometric Function1/1
  Trigonometric Function/1 -> Create 2x2 Matrix/1(A00), Create 2x2 Matrix/4(A11)
  Trigonometric Function1/1 -> Create 2x2 Matrix/2(A01), Gain/1

== system UserVehicle_RTW/UserVehicle/Single Track Model/vehicle motion/global frame/Calc_Tr2Fr0_2D/Create 2x2 Matrix ==
  A00 : Inport
  A01 : Inport  Port=2
  A10 : Inport  Port=3
  A11 : Inport  Port=4
  Matrix Concatenate : Concatenate  Mode=Multidimensional array
  Matrix Concatenate1 : Concatenate  Mode=Multidimensional array  ConcatenateDimension=2
  Matrix Concatenate2 : Concatenate  Mode=Multidimensional array  ConcatenateDimension=2
  A : Outport  VectorParamsAs1DForOutWhenUnconnected=off
  wires:
  Matrix Concatenate1/1 -> Matrix Concatenate/1
  A00/1 -> Matrix Concatenate1/1
  A01/1 -> Matrix Concatenate1/2
  Matrix Concatenate2/1 -> Matrix Concatenate/2
  A10/1 -> Matrix Concatenate2/1
  A11/1 -> Matrix Concatenate2/2
  Matrix Concatenate/1 -> A/1

== system UserVehicle_RTW/UserVehicle/Single Track Model/vehicle motion/vehicle frame/Car.vx_1/PassIfSim ==
  note: Output original value only when simulating,
      | and zero during pre- or postprocessing.
  In1 : Inport
  "   " : Product  InputSameDT=on  SaturateOnIntegerOverflow=on  OutDataTypeStr=Inherit: Same as first input
  Data Type Conversion : DataTypeConversion
  Out1 : Outport  VectorParamsAs1DForOutWhenUnconnected=off
  wires:
  In1/1 -> "   "/1
  Data Type Conversion/1 -> "   "/2
  "   "/1 -> Out1/1
  [TRSim] -> Data Type Conversion/1

== system UserVehicle_RTW/UserVehicle/Single Track Model/tire forces/contact point velocities/front/Calc_Tr2FrW_2D/Create 2x2 Matrix ==
  A00 : Inport
  A01 : Inport  Port=2
  A10 : Inport  Port=3
  A11 : Inport  Port=4
  Matrix Concatenate : Concatenate  Mode=Multidimensional array
  Matrix Concatenate1 : Concatenate  Mode=Multidimensional array  ConcatenateDimension=2
  Matrix Concatenate2 : Concatenate  Mode=Multidimensional array  ConcatenateDimension=2
  A : Outport  VectorParamsAs1DForOutWhenUnconnected=off
  wires:
  Matrix Concatenate1/1 -> Matrix Concatenate/1
  A00/1 -> Matrix Concatenate1/1
  A01/1 -> Matrix Concatenate1/2
  Matrix Concatenate2/1 -> Matrix Concatenate/2
  A10/1 -> Matrix Concatenate2/1
  A11/1 -> Matrix Concatenate2/2
  Matrix Concatenate/1 -> A/1
